simulink model "AUAV3_AND_SLUGS_SENSOR"  (Simulink 7.8)
settings: Solver=FixedStepDiscrete  StartTime=0.0  StopTime=10.0  FixedStep=T  RelTol=1e-3
PreLoadFcn:
  | T = 0.0025;
  | MavlinkBus;
  | 
  | % Baro Altitude Computation
  | % =========================
  | basePressure = 98192.64;
  | baseTemp = 288.215;
  | lapseRate = -0.00198122;
  | baseHeight = 0;
  | 
  | mcuInit
values from neighbouring files (symbols this model uses):
  apSampleTime = 0.01    [mcuInit.m]
  mavlink_gps_raw_int_t = Simulink.Bus    [MavlinkBus.m]    (also in MavlinkBusMarcello.m)
  mavlink_raw_imu_t = Simulink.Bus    [MavlinkBus.m]    (also in MavlinkBusMarcello.m)
  mavlink_scaled_pressure_t = Simulink.Bus    [MavlinkBus.m]    (also in MavlinkBusMarcello.m)
  mavlink_sys_status_t = Simulink.Bus    [MavlinkBus.m]    (also in MavlinkBusMarcello.m)
undefined symbols (not defined in the file or in its folder): A0, A14, A15, A2, A3, A5, A6, B0, barAdjust, baroCutTemp, baroOffset, baroScale, barTGain1, barTGain2, barTMean1, barTMean2, cubeAccelGain16405, cubeGyroGain16405, cubeMagGain16405, D0, D11, D8, G0, G15, gaind, IC1max, lowRateSensorCutoff, mainSensorCutoff, Max, maxDynPressure, ms, OC1max, P112, P127, P16, P21, P30, P31, P64, P72, P75, P80, P82, P83, Pin, pitAdjust, pitCutTemp, pitotOffset, pitotScale, pitTGain1, pitTGain2, pitTMean1, pitTMean2, polesd, powerOffset, powerScale, pressureSensorCutoff, Resol, tempOffset, tempScale ... (+5)
libraries: MCHP_Blockset x56, simulink x21, aerolibconvert2 x2
(part 4 of 5)

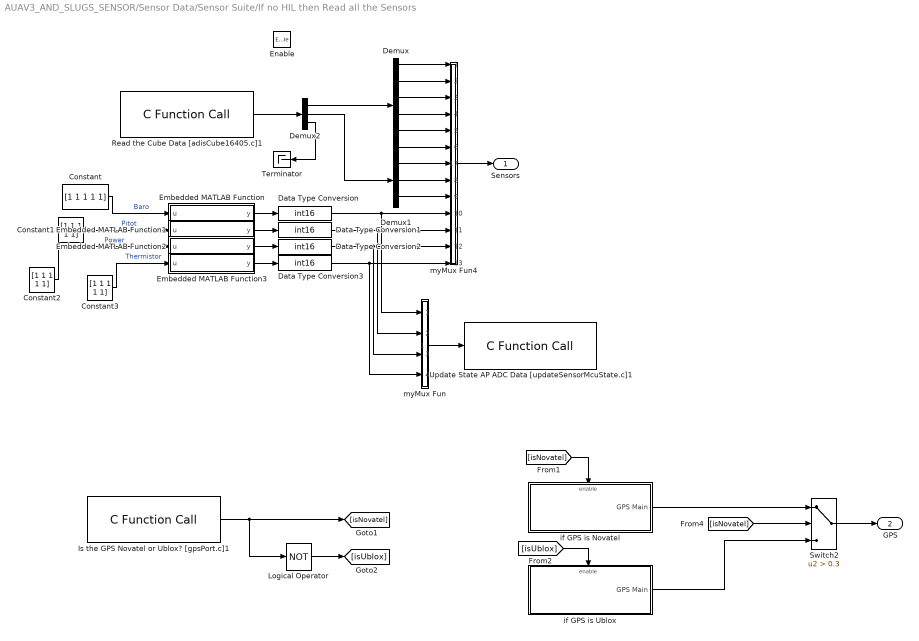
== system AUAV3_AND_SLUGS_SENSOR/Sensor Data/Sensor Suite/If no HIL then Read all the Sensors ==
  Enable : EnablePort
  Constant{,1..3} (4 alike) : Constant  Value=[1 1 1 1 1]
  Data Type Conversion{,1..3} (4 alike) : DataTypeConversion  OutDataTypeStr=int16
  Demux : Demux  Outputs=6
  Demux1 : Demux  Outputs=3
  Demux2 : Demux  Outputs=[6 3 1]
  Embedded MATLAB Function : MATLAB Function  TreatAsAtomicUnit=on
  Embedded MATLAB Function1 : MATLAB Function  TreatAsAtomicUnit=on
  Embedded MATLAB Function2 : MATLAB Function  TreatAsAtomicUnit=on
  Embedded MATLAB Function3 : MATLAB Function  TreatAsAtomicUnit=on
  Is the GPS Novatel or Ublox? [gpsPort.c]1 : MCHP_Blockset/User Functions/C Function Call  ParseFilesChkbx=off  ListFunctions1=Custom Function  Function1=extern uint8_T isGPSNovatel();  AddHeaderDeclaration=off  Function1Type=when block is updated (default)  FctReturnBlockOut=off  Fct1BlockOut=y[2]  DataCollected=0  ORDERING=Output  SampleTime=.01  MCHP_MASTERLINK=|  PinDigitalInput=[]  PinDigitalOutput=[]  PinAnalogInput=[]
      | AUAV3_AND_SLUGS_SENSOR/Microchip Master
      | AUAV V3 Board
      | Busy Flag on D2 (RA6)
  Logical Operator : Logic  Operator=NOT  AllPortsSameDT=off  OutDataTypeStr=boolean
  Read the Cube Data [adisCube16405.c]1 : MCHP_Blockset/User Functions/C Function Call  ParseFilesChkbx=off  ListFunctions1=Custom Function  Function1=extern void getCubeData(int16_T* y1);  AddHeaderDeclaration=off  Function1Type=when block is updated (default)  FctReturnBlockOut=off  Fct1BlockOut=y1[10]  ORDERING=None  SampleTime=.01  MCHP_MASTERLINK=|  PinDigitalInput=[]  PinDigitalOutput=[]  PinAnalogInput=[]
      | AUAV3_AND_SLUGS_SENSOR/Microchip Master
      | AUAV V3 Board
      | Busy Flag on D2 (RA6)
  Switch2 : Switch  Criteria=u2 > Threshold  Threshold=0.3  ZeroCross=off
  Terminator : Terminator
  Update State AP ADC Data [updateSensorMcuState.c]1 : MCHP_Blockset/User Functions/C Function Call  ParseFilesChkbx=off  ListFunctions1=Custom Function  Function1=extern void updateRawADCData(int16_T* u1);  AddHeaderDeclaration=off  Function1Type=when block is updated (default)  Fct1BlockIn=u1  FctReturnBlockOut=off  Fct1BlockOut=u1  DataCollected=0  ORDERING=None  SampleTime=.01  MCHP_MASTERLINK=|  PinDigitalInput=[]  PinDigitalOutput=[]  PinAnalogInput=[]
      | AUAV3_AND_SLUGS_SENSOR/Microchip Master
      | AUAV V3 Board
      | Busy Flag on D2 (RA6)
  if GPS is Novatel : Subsystem
  if GPS is Ublox : Subsystem
  myMux Fun : MATLAB Function  TreatAsAtomicUnit=on
  myMux Fun4 : MATLAB Function  TreatAsAtomicUnit=on
  Sensors : Outport
  GPS : Outport  Port=2
  wires:
  myMux Fun4/1(y) -> Sensors/1
  Demux2/1 -> Demux/1
  Demux/1 -> myMux Fun4/1(u1)
  Demux/2 -> myMux Fun4/2(u2)
  Demux/3 -> myMux Fun4/3(u3)
  Demux/4 -> myMux Fun4/4(u4)
  Demux/5 -> myMux Fun4/5(u5)
  Demux/6 -> myMux Fun4/6(u6)
  Demux1/1 -> myMux Fun4/7(u7)
  Demux1/2 -> myMux Fun4/8(u8)
  Demux1/3 -> myMux Fun4/9(u9)
  Constant/1 -> Embedded MATLAB Function/1(u)  "Baro"
  Constant1/1 -> Embedded MATLAB Function1/1(u)  "Pitot"
  Constant2/1 -> Embedded MATLAB Function2/1(u)  "Power"
  Constant3/1 -> Embedded MATLAB Function3/1(u)  "Thermistor"
  myMux Fun/1(y) -> Update State AP ADC Data [updateSensorMcuState.c]1/1
  Data Type Conversion/1 -> myMux Fun4/10(u10), myMux Fun/1(u1)
  Data Type Conversion1/1 -> myMux Fun4/11(u11), myMux Fun/2(u2)
  Data Type Conversion2/1 -> myMux Fun4/12(u12), myMux Fun/3(u3)
  Data Type Conversion3/1 -> myMux Fun4/13(u13), myMux Fun/4(u4)
  Embedded MATLAB Function/1(y) -> Data Type Conversion/1
  Embedded MATLAB Function1/1(y) -> Data Type Conversion1/1
  Embedded MATLAB Function2/1(y) -> Data Type Conversion2/1
  Embedded MATLAB Function3/1(y) -> Data Type Conversion3/1
  Read the Cube Data [adisCube16405.c]1/1 -> Demux2/1
  Demux2/3 -> Terminator/1
  Demux2/2 -> Demux1/1
  [isNovatel] -> Switch2/2
  Switch2/1 -> GPS/1
  Is the GPS Novatel or Ublox? [gpsPort.c]1/1 -> [isNovatel], Logical Operator/1
  if GPS is Novatel/1(GPS Main) -> Switch2/1
  Logical Operator/1 -> [isUblox]
  [isNovatel] -> if GPS is Novatel/Enable
  [isUblox] -> if GPS is Ublox/Enable
  if GPS is Ublox/1(GPS Main) -> Switch2/3

== system AUAV3_AND_SLUGS_SENSOR/Sensor Data/Sensor Suite/If no HIL then update Air Data ==
  AirData : Inport
  Enable : EnablePort
  Demux : Demux  Outputs=[1 2]
  Terminator : Terminator
  Update the Air Calibrated Data [updateSensorMcuState.c]1 : MCHP_Blockset/User Functions/C Function Call  ParseFilesChkbx=off  ListFunctions1=Custom Function  Function1=extern void updateAirData(real32_T* u1);  AddHeaderDeclaration=off  Function1Type=when block is updated (default)  FctReturnBlockOut=off  DataCollected=0  ORDERING=None  SampleTime=.01  MCHP_MASTERLINK=|  PinDigitalInput=[]  PinDigitalOutput=[]  PinAnalogInput=[]
      | AUAV3_AND_SLUGS_SENSOR/Microchip Master
      | AUAV V3 Board
      | Busy Flag on D2 (RA6)
  Out1 : Outport
  wires:
  AirData/1 -> Demux/1, Update the Air Calibrated Data [updateSensorMcuState.c]1/1
  Demux/1 -> Out1/1
  Demux/2 -> Terminator/1

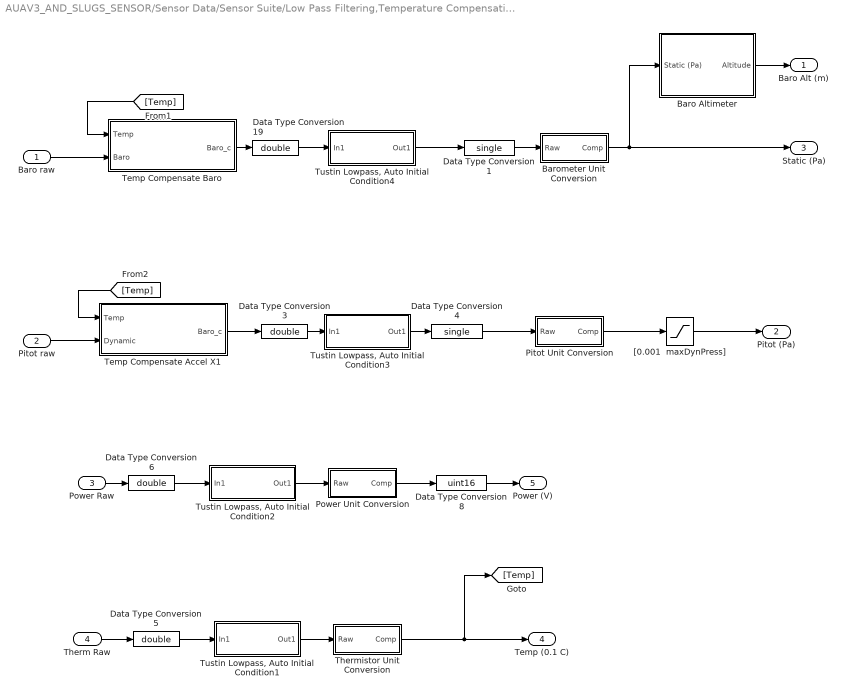
== system AUAV3_AND_SLUGS_SENSOR/Sensor Data/Sensor Suite/Low Pass Filtering,Temperature Compensation and Calibration ==
  Baro raw : Inport
  Pitot raw : Inport  Port=2
  Power Raw : Inport  Port=3
  Therm Raw : Inport  Port=4
  Baro Altimeter : Subsystem
  Barometer Unit Conversion : Subsystem  mask{bias=baroOffset, gains=baroScale}
      mask prompts: bias "Initial Bias"; gains "Initial Gains"
      mask help: Convert Analog readings to units
  Data Type Conversion1 : DataTypeConversion  OutDataTypeStr=single
  Data Type Conversion{3,5..6,19} (4 alike) : DataTypeConversion  OutDataTypeStr=double
  Data Type Conversion4 : DataTypeConversion  OutDataTypeStr=single
  Data Type Conversion8 : DataTypeConversion  OutDataTypeStr=uint16
  Pitot Unit Conversion : Subsystem  mask{bias=pitotOffset, gains=pitotScale}
      mask prompts: bias "Initial Bias"; gains "Initial Gains"
      mask help: Convert Analog readings to units
  Power Unit Conversion : Subsystem  mask{bias=powerOffset, gains=powerScale}
      mask prompts: bias "Initial Bias"; gains "Initial Gains"
      mask help: Convert Analog readings to units
  Temp Compensate Accel X1 : Subsystem
  Temp Compensate Baro : Subsystem
  Thermistor Unit Conversion : Subsystem  mask{bias=tempOffset, gains=tempScale}
      mask prompts: bias "Initial Bias"; gains "Initial Gains"
      mask help: Convert Analog readings to units
  "Tustin Lowpass, Auto Initial Condition1" : Subsystem  mask(Tustin1stOrderLowpassAutoInitialCondition){f=lowRateSensorCutoff, T=apSampleTime}
      mask prompts: f "Lowpass Frequency"; T "Sample Time"
      mask help: Takes a 3db rolloff frequency (in Hz, NOT radians/s) and a sample time. Performs a symbolic Tustin conversion and implements in a discrete filter. The initial output of the filter is set by the first sample.
      mask Help: Enter the desired 3db rolloff frequency in Hz and the sample time. Initial conditions are sampled automatically.
      mask Display: fprintf('%.2f Hz lowpass',f)
  "Tustin Lowpass, Auto Initial Condition2" : Subsystem  mask(Tustin1stOrderLowpassAutoInitialCondition){f=lowRateSensorCutoff, T=apSampleTime}
      mask prompts: f "Lowpass Frequency"; T "Sample Time"
      mask help: Takes a 3db rolloff frequency (in Hz, NOT radians/s) and a sample time. Performs a symbolic Tustin conversion and implements in a discrete filter. The initial output of the filter is set by the first sample.
      mask Help: Enter the desired 3db rolloff frequency in Hz and the sample time. Initial conditions are sampled automatically.
      mask Display: fprintf('%.2f Hz lowpass',f)
  "Tustin Lowpass, Auto Initial Condition3" : Subsystem  mask(Tustin1stOrderLowpassAutoInitialCondition){f=pressureSensorCutoff, T=apSampleTime}
      mask prompts: f "Lowpass Frequency"; T "Sample Time"
      mask help: Takes a 3db rolloff frequency (in Hz, NOT radians/s) and a sample time. Performs a symbolic Tustin conversion and implements in a discrete filter. The initial output of the filter is set by the first sample.
      mask Help: Enter the desired 3db rolloff frequency in Hz and the sample time. Initial conditions are sampled automatically.
      mask Display: fprintf('%.2f Hz lowpass',f)
  "Tustin Lowpass, Auto Initial Condition4" : Subsystem  mask(Tustin1stOrderLowpassAutoInitialCondition){f=pressureSensorCutoff, T=apSampleTime}
      mask prompts: f "Lowpass Frequency"; T "Sample Time"
      mask help: Takes a 3db rolloff frequency (in Hz, NOT radians/s) and a sample time. Performs a symbolic Tustin conversion and implements in a discrete filter. The initial output of the filter is set by the first sample.
      mask Help: Enter the desired 3db rolloff frequency in Hz and the sample time. Initial conditions are sampled automatically.
      mask Display: fprintf('%.2f Hz lowpass',f)
  "[0.001  maxDynPress]" : Saturate  UpperLimit=maxDynPressure  LowerLimit=0.001
  Baro Alt (m) : Outport
  Pitot (Pa) : Outport  Port=2
  Static (Pa) : Outport  Port=3
  Temp (0.1 C) : Outport  Port=4
  Power (V) : Outport  Port=5
  wires:
  "Tustin Lowpass, Auto Initial Condition1"/1(Out1) -> Thermistor Unit Conversion/1(Raw)
  "[0.001  maxDynPress]"/1 -> Pitot (Pa)/1
  Data Type Conversion19/1 -> "Tustin Lowpass, Auto Initial Condition4"/1(In1)
  Data Type Conversion3/1 -> "Tustin Lowpass, Auto Initial Condition3"/1(In1)
  "Tustin Lowpass, Auto Initial Condition3"/1(Out1) -> Data Type Conversion4/1
  Data Type Conversion5/1 -> "Tustin Lowpass, Auto Initial Condition1"/1(In1)
  Therm Raw/1 -> Data Type Conversion5/1
  Barometer Unit Conversion/1(Comp) -> Static (Pa)/1, Baro Altimeter/1(Static (Pa))
  Data Type Conversion4/1 -> Pitot Unit Conversion/1(Raw)
  "Tustin Lowpass, Auto Initial Condition4"/1(Out1) -> Data Type Conversion1/1
  Data Type Conversion1/1 -> Barometer Unit Conversion/1(Raw)
  Thermistor Unit Conversion/1(Comp) -> Temp (0.1 C)/1, [Temp]
  Data Type Conversion6/1 -> "Tustin Lowpass, Auto Initial Condition2"/1(In1)
  Power Raw/1 -> Data Type Conversion6/1
  "Tustin Lowpass, Auto Initial Condition2"/1(Out1) -> Power Unit Conversion/1(Raw)
  Data Type Conversion8/1 -> Power (V)/1
  Baro Altimeter/1(Altitude) -> Baro Alt (m)/1
  Pitot Unit Conversion/1(Comp) -> "[0.001  maxDynPress]"/1
  Power Unit Conversion/1(Comp) -> Data Type Conversion8/1
  Temp Compensate Baro/1(Baro_c) -> Data Type Conversion19/1
  [Temp] -> Temp Compensate Baro/1(Temp)
  Baro raw/1 -> Temp Compensate Baro/2(Baro)
  [Temp] -> Temp Compensate Accel X1/1(Temp)
  Pitot raw/1 -> Temp Compensate Accel X1/2(Dynamic)
  Temp Compensate Accel X1/1(Baro_c) -> Data Type Conversion3/1

== system AUAV3_AND_SLUGS_SENSOR/Read Barometer BMP180/Baro Altimeter/Initial Baro Bias/Low Pass8 ==
  In1 : Inport
  Discrete Zero-Pole : DiscreteZeroPole  Zeros=zerosd  Poles=polesd  Gain=gaind  SampleTime=SampleTime
  Out1 : Outport
  wires:
  Discrete Zero-Pole/1 -> Out1/1
  In1/1 -> Discrete Zero-Pole/1

== system AUAV3_AND_SLUGS_SENSOR/Sensor Data/Sensor Suite/ADIS16405 Signal Cond /3D Tustin Lowpass, Auto Initial Condition ==
  In1 : Inport
  Constant : Constant  Value=T
  Constant1 : Constant  Value=f
  Constant2 : Constant  Value=T
  Constant3 : Constant  Value=f
  Constant4 : Constant  Value=T
  Constant5 : Constant  Value=f
  Demux : Demux  Outputs=3
  Embedded MATLAB Function : MATLAB Function  TreatAsAtomicUnit=on
  Embedded MATLAB Function1 : MATLAB Function  TreatAsAtomicUnit=on
  Embedded MATLAB Function2 : MATLAB Function  TreatAsAtomicUnit=on
  myMux Fun : MATLAB Function  TreatAsAtomicUnit=on
  Out1 : Outport
  wires:
  myMux Fun/1(y) -> Out1/1
  In1/1 -> Demux/1
  Embedded MATLAB Function1/1(y) -> myMux Fun/2(u2)
  Demux/3 -> Embedded MATLAB Function2/1(u)
  Demux/2 -> Embedded MATLAB Function1/1(u)
  Demux/1 -> Embedded MATLAB Function/1(u)
  Embedded MATLAB Function2/1(y) -> myMux Fun/3(u3)
  Constant5/1 -> Embedded MATLAB Function2/3(f)
  Constant4/1 -> Embedded MATLAB Function2/2(T)
  Constant3/1 -> Embedded MATLAB Function1/3(f)
  Constant2/1 -> Embedded MATLAB Function1/2(T)
  Embedded MATLAB Function/1(y) -> myMux Fun/1(u1)
  Constant1/1 -> Embedded MATLAB Function/3(f)
  Constant/1 -> Embedded MATLAB Function/2(T)

== system AUAV3_AND_SLUGS_SENSOR/Sensor Data/Sensor Suite/ADIS16405 Signal Cond /3D Tustin Lowpass, Auto Initial Condition1 ==
  In1 : Inport
  Constant : Constant  Value=T
  Constant1 : Constant  Value=f
  Constant2 : Constant  Value=T
  Constant3 : Constant  Value=f
  Constant4 : Constant  Value=T
  Constant5 : Constant  Value=f
  Demux : Demux  Outputs=3
  Embedded MATLAB Function : MATLAB Function  TreatAsAtomicUnit=on
  Embedded MATLAB Function1 : MATLAB Function  TreatAsAtomicUnit=on
  Embedded MATLAB Function2 : MATLAB Function  TreatAsAtomicUnit=on
  myMux Fun : MATLAB Function  TreatAsAtomicUnit=on
  Out1 : Outport
  wires:
  myMux Fun/1(y) -> Out1/1
  In1/1 -> Demux/1
  Embedded MATLAB Function1/1(y) -> myMux Fun/2(u2)
  Demux/3 -> Embedded MATLAB Function2/1(u)
  Demux/2 -> Embedded MATLAB Function1/1(u)
  Demux/1 -> Embedded MATLAB Function/1(u)
  Embedded MATLAB Function2/1(y) -> myMux Fun/3(u3)
  Constant5/1 -> Embedded MATLAB Function2/3(f)
  Constant4/1 -> Embedded MATLAB Function2/2(T)
  Constant3/1 -> Embedded MATLAB Function1/3(f)
  Constant2/1 -> Embedded MATLAB Function1/2(T)
  Embedded MATLAB Function/1(y) -> myMux Fun/1(u1)
  Constant1/1 -> Embedded MATLAB Function/3(f)
  Constant/1 -> Embedded MATLAB Function/2(T)

== system AUAV3_AND_SLUGS_SENSOR/Sensor Data/Sensor Suite/ADIS16405 Signal Cond /3D Tustin Lowpass, Auto Initial Condition2 ==
  In1 : Inport
  Constant : Constant  Value=T
  Constant1 : Constant  Value=f
  Constant2 : Constant  Value=T
  Constant3 : Constant  Value=f
  Constant4 : Constant  Value=T
  Constant5 : Constant  Value=f
  Demux : Demux  Outputs=3
  Embedded MATLAB Function : MATLAB Function  TreatAsAtomicUnit=on
  Embedded MATLAB Function1 : MATLAB Function  TreatAsAtomicUnit=on
  Embedded MATLAB Function2 : MATLAB Function  TreatAsAtomicUnit=on
  myMux Fun : MATLAB Function  TreatAsAtomicUnit=on
  Out1 : Outport
  wires:
  Constant/1 -> Embedded MATLAB Function/2(T)
  Constant1/1 -> Embedded MATLAB Function/3(f)
  Embedded MATLAB Function/1(y) -> myMux Fun/1(u1)
  Constant2/1 -> Embedded MATLAB Function1/2(T)
  Constant3/1 -> Embedded MATLAB Function1/3(f)
  Constant4/1 -> Embedded MATLAB Function2/2(T)
  Constant5/1 -> Embedded MATLAB Function2/3(f)
  Embedded MATLAB Function2/1(y) -> myMux Fun/3(u3)
  Demux/1 -> Embedded MATLAB Function/1(u)
  Demux/2 -> Embedded MATLAB Function1/1(u)
  Demux/3 -> Embedded MATLAB Function2/1(u)
  Embedded MATLAB Function1/1(y) -> myMux Fun/2(u2)
  In1/1 -> Demux/1
  myMux Fun/1(y) -> Out1/1

== system AUAV3_AND_SLUGS_SENSOR/Sensor Data/Sensor Suite/ADIS16405 Signal Cond /Rotate Cube Axis ==
  Raw : Inport
  Selector : Selector  InputPortWidth=3  IndexOptions=Index vector (dialog)  Indices=[2 1 3]  OutputSizes=1
  "[ -1 -1 -1]" : Gain  Gain=[-1 -1 -1]
  Rotated : Outport
  wires:
  Selector/1 -> "[ -1 -1 -1]"/1
  Raw/1 -> Selector/1
  "[ -1 -1 -1]"/1 -> Rotated/1

== system AUAV3_AND_SLUGS_SENSOR/Sensor Data/Sensor Suite/ADIS16405 Signal Cond /Rotate Cube Axis  ==
  Raw : Inport
  Selector : Selector  InputPortWidth=3  IndexOptions=Index vector (dialog)  Indices=[2 1 3]  OutputSizes=1
  Rotated : Outport
  wires:
  Raw/1 -> Selector/1
  Selector/1 -> Rotated/1

== system AUAV3_AND_SLUGS_SENSOR/Sensor Data/Sensor Suite/ADIS16405 Signal Cond /Rotate Cube Axis   ==
  Raw : Inport
  Selector : Selector  InputPortWidth=3  IndexOptions=Index vector (dialog)  Indices=[2 1 3]  OutputSizes=1
  "[ -1 -1 -1]" : Gain  Gain=[-1 -1 -1]
  Rotated : Outport
  wires:
  "[ -1 -1 -1]"/1 -> Rotated/1
  Raw/1 -> Selector/1
  Selector/1 -> "[ -1 -1 -1]"/1

== system AUAV3_AND_SLUGS_SENSOR/Sensor Data/Sensor Suite/If no HIL then Read all the Sensors/if GPS is Novatel ==
  Enable : EnablePort
  Parse the GPS RAW Data [gps.c/novatel.c]1 : MCHP_Blockset/User Functions/C Function Call  ParseFilesChkbx=off  ListFunctions1=Custom Function  Function1=extern void gpsParse(uint8_T* u1);  AddHeaderDeclaration=off  Function1Type=when block is updated (default)  Fct1BlockIn=u1  FctReturnBlockOut=off  Fct1BlockOut=u1*  DataCollected=0  ORDERING=None  SampleTime=.01  MCHP_MASTERLINK=|  PinDigitalInput=[]  PinDigitalOutput=[]  PinAnalogInput=[]
      | AUAV3_AND_SLUGS_SENSOR/Microchip Master
      | AUAV V3 Board
      | Busy Flag on D2 (RA6)
  Produce the GPS Main Data and update the AP State (lat lon hei cog sog) [gps.c/novatel.c]1 : MCHP_Blockset/User Functions/C Function Call  ParseFilesChkbx=off  ListFunctions1=Custom Function  Function1=extern void getGpsMainData(real32_T* y1);  AddHeaderDeclaration=off  Function1Type=when block is updated (default)  FctReturnBlockOut=off  Fct1BlockOut=y1  DataCollected=0  ORDERING=None  SampleTime=.01  MCHP_MASTERLINK=|  PinDigitalInput=[]  PinDigitalOutput=[]  PinAnalogInput=[]
      | AUAV3_AND_SLUGS_SENSOR/Microchip Master
      | AUAV V3 Board
      | Busy Flag on D2 (RA6)
  Read the Raw Data from GPS [gpsPort.c]1 : MCHP_Blockset/User Functions/C Function Call  ParseFilesChkbx=off  ListFunctions1=Custom Function  Function1=extern void getGPSRawData(uint8_T* y1);  AddHeaderDeclaration=off  Function1Type=when block is updated (default)  FctReturnBlockOut=off  Fct1BlockOut=y1  DataCollected=0  ORDERING=None  SampleTime=.01  MCHP_MASTERLINK=|  PinDigitalInput=[]  PinDigitalOutput=[]  PinAnalogInput=[]
      | AUAV3_AND_SLUGS_SENSOR/Microchip Master
      | AUAV V3 Board
      | Busy Flag on D2 (RA6)
  GPS Main : Outport
  wires:
  Produce the GPS Main Data and update the AP State (lat lon hei cog sog) [gps.c/novatel.c]1/1 -> GPS Main/1
  Read the Raw Data from GPS [gpsPort.c]1/1 -> Parse the GPS RAW Data [gps.c/novatel.c]1/1

== system AUAV3_AND_SLUGS_SENSOR/Sensor Data/Sensor Suite/If no HIL then Read all the Sensors/if GPS is Ublox ==
  Enable : EnablePort
  Produce the GPS Main Data and update the AP State (lat lon hei cog sog) [gpsUblox.c]1 : MCHP_Blockset/User Functions/C Function Call  ParseFilesChkbx=off  ListFunctions1=Custom Function  Function1=extern void getGpsUbloxMainData(real32_T* y1);  AddHeaderDeclaration=off  Function1Type=when block is updated (default)  FctReturnBlockOut=off  Fct1BlockOut=y1  DataCollected=0  ORDERING=None  SampleTime=.01  MCHP_MASTERLINK=|  PinDigitalInput=[]  PinDigitalOutput=[]  PinAnalogInput=[]
      | AUAV3_AND_SLUGS_SENSOR/Microchip Master
      | AUAV V3 Board
      | Busy Flag on D2 (RA6)
  GPS Main : Outport
  wires:
  Produce the GPS Main Data and update the AP State (lat lon hei cog sog) [gpsUblox.c]1/1 -> GPS Main/1

== system AUAV3_AND_SLUGS_SENSOR/Sensor Data/Sensor Suite/Low Pass Filtering,Temperature Compensation and Calibration/Baro Altimeter ==
  Static (Pa) : Inport
  Compute Barometric Height : Subsystem  mask{baseTemp=baseTemp, LapseRate=lapseRate}
      mask prompts: baseTemp "Base Station Temperature (K)"; LapseRate "Lapse Rate (C/ft)"
      mask help:
      | Produces Altitude in meters from Barometric Pressure in Pascals. Altitude is valid from MSL to 6000 ft.
      |
      | The method implemented here was developed by Ren Curry
  Enabled Subsystem : Subsystem  TreatAsAtomicUnit=on
  Enables/Disables the Computation of  initial Baro Bias : MATLAB Function  TreatAsAtomicUnit=on
  GS Height : Subsystem
  Initial Baro Bias : Subsystem  TreatAsAtomicUnit=on
  Logical Operator : Logic  Operator=NOT  AllPortsSameDT=off  OutDataTypeStr=boolean
  Sum1 : Sum  Inputs=++|  OutDataTypeStr=single
  Zero Out Height : Subsystem  TreatAsAtomicUnit=on
  Altitude : Outport
  wires:
  Compute Barometric Height/1("Altitude, m") -> Zero Out Height/2(Computed Height), Sum1/2
  Static (Pa)/1 -> Initial Baro Bias/1(Baro (Pa)), Compute Barometric Height/3(Baro (Pa))
  Enables/Disables the Computation of  initial Baro Bias/1(tOut) -> Initial Baro Bias/Enable, Zero Out Height/Enable, Logical Operator/1
  GS Height/1(GS Height) -> Compute Barometric Height/1(Base Height (m)), Zero Out Height/1(Base Height)
  Initial Baro Bias/1(Baro (Gnd)) -> Compute Barometric Height/2(Base Pressure (Pa))
  Zero Out Height/1(Height Offset) -> Sum1/1
  Logical Operator/1 -> Enabled Subsystem/Enable
  Sum1/1 -> Enabled Subsystem/1(In1)
  Enabled Subsystem/1(Out1) -> Altitude/1

== system AUAV3_AND_SLUGS_SENSOR/Sensor Data/Sensor Suite/Low Pass Filtering,Temperature Compensation and Calibration/Barometer Unit Conversion ==
  Raw : Inport
  Bias : Constant  Value=bias  OutDataTypeStr=single
  Divide : Product  OutDataTypeStr=single
  Gains : Constant  Value=gains  OutDataTypeStr=single
  Sum : Sum  Inputs=|++  OutDataTypeStr=single
  Comp : Outport
  wires:
  Bias/1 -> Sum/2
  Raw/1 -> Divide/2
  Gains/1 -> Divide/1
  Divide/1 -> Sum/1
  Sum/1 -> Comp/1

== system AUAV3_AND_SLUGS_SENSOR/Sensor Data/Sensor Suite/Low Pass Filtering,Temperature Compensation and Calibration/Pitot Unit Conversion ==
  Raw : Inport
  Bias : Constant  Value=bias  OutDataTypeStr=single
  Divide : Product  OutDataTypeStr=single
  Gains : Constant  Value=gains  OutDataTypeStr=single
  Sum : Sum  Inputs=|++  OutDataTypeStr=single
  Comp : Outport
  wires:
  Bias/1 -> Sum/2
  Raw/1 -> Divide/2
  Gains/1 -> Divide/1
  Divide/1 -> Sum/1
  Sum/1 -> Comp/1

== system AUAV3_AND_SLUGS_SENSOR/Sensor Data/Sensor Suite/Low Pass Filtering,Temperature Compensation and Calibration/Power Unit Conversion ==
  Raw : Inport
  Bias : Constant  Value=bias  OutDataTypeStr=single
  Divide : Product  OutDataTypeStr=single
  Gains : Constant  Value=gains  OutDataTypeStr=single
  Sum : Sum  Inputs=|++  OutDataTypeStr=single
  Comp : Outport
  wires:
  Bias/1 -> Sum/2
  Raw/1 -> Divide/2
  Gains/1 -> Divide/1
  Divide/1 -> Sum/1
  Sum/1 -> Comp/1

== system AUAV3_AND_SLUGS_SENSOR/Sensor Data/Sensor Suite/Low Pass Filtering,Temperature Compensation and Calibration/Temp Compensate Accel X1 ==
  Temp : Inport
  Dynamic : Inport  Port=2
  Compare To Constant : simulink/Logic and Bit Operations/Compare To Constant  relop=<  const=pitCutTemp  OutDataTypeStr=uint8  ZeroCross=off
  Display : Display
  Display2 : Display
  Hi Temp Compensation2 : Subsystem  mask{alpha=pitTGain2, tempMean=pitTMean2}
      mask prompts: alpha "Tempearature Coeficient (K_t)"; tempMean "Calibration Temperature Mean (T_avg)"
      mask help:
      | This block implements a temperature compensation. It implmements the following equation:
      |
      | M_tc = M_raw - K_t(T - T_avg)
  Lo Temp Compensation : Subsystem  mask{alpha=pitTGain1, tempMean=pitTMean1}
      mask prompts: alpha "Tempearature Coeficient (K_t)"; tempMean "Calibration Temperature Mean (T_avg)"
      mask help:
      | This block implements a temperature compensation. It implmements the following equation:
      |
      | M_tc = M_raw - K_t(T - T_avg)
  Logical Operator : Logic  Operator=NOT  AllPortsSameDT=off  OutDataTypeStr=boolean
  Merge : Merge
  Baro_c : Outport
  wires:
  Hi Temp Compensation2/1(Comp) -> Merge/1
  Logical Operator/1 -> Hi Temp Compensation2/Enable, Display2/1
  Merge/1 -> Baro_c/1, Display/1
  Dynamic/1 -> Lo Temp Compensation/1(Raw), Hi Temp Compensation2/1(Raw)
  Temp/1 -> Compare To Constant/1, Lo Temp Compensation/2(Temp Raw), Hi Temp Compensation2/2(Temp Raw)
  Compare To Constant/1 -> Lo Temp Compensation/Enable, Logical Operator/1
  Lo Temp Compensation/1(Comp) -> Merge/2

== system AUAV3_AND_SLUGS_SENSOR/Sensor Data/Sensor Suite/Low Pass Filtering,Temperature Compensation and Calibration/Temp Compensate Baro ==
  Temp : Inport
  Baro : Inport  Port=2
  Compare To Constant : simulink/Logic and Bit Operations/Compare To Constant  relop=<  const=baroCutTemp  OutDataTypeStr=uint8  ZeroCross=off
  Hi Temp Compensation : Subsystem  mask{alpha=barTGain2, tempMean=barTMean2}
      mask prompts: alpha "Tempearature Coeficient (K_t)"; tempMean "Calibration Temperature Mean (T_avg)"
      mask help:
      | This block implements a temperature compensation. It implmements the following equation:
      |
      | M_tc = M_raw - K_t(T - T_avg)
  Lo Temp Compensation : Subsystem  mask{alpha=barTGain1, tempMean=barTMean1}
      mask prompts: alpha "Tempearature Coeficient (K_t)"; tempMean "Calibration Temperature Mean (T_avg)"
      mask help:
      | This block implements a temperature compensation. It implmements the following equation:
      |
      | M_tc = M_raw - K_t(T - T_avg)
  Logical Operator : Logic  Operator=NOT  AllPortsSameDT=off  OutDataTypeStr=boolean
  Merge : Merge
  Baro_c : Outport
  wires:
  Compare To Constant/1 -> Logical Operator/1, Lo Temp Compensation/Enable
  Temp/1 -> Compare To Constant/1, Hi Temp Compensation/2(Temp Raw), Lo Temp Compensation/2(Temp Raw)
  Baro/1 -> Hi Temp Compensation/1(Raw), Lo Temp Compensation/1(Raw)
  Lo Temp Compensation/1(Comp) -> Merge/2
  Merge/1 -> Baro_c/1
  Logical Operator/1 -> Hi Temp Compensation/Enable
  Hi Temp Compensation/1(Comp) -> Merge/1

== system AUAV3_AND_SLUGS_SENSOR/Sensor Data/Sensor Suite/Low Pass Filtering,Temperature Compensation and Calibration/Thermistor Unit Conversion ==
  Raw : Inport
  Bias : Constant  Value=bias  OutDataTypeStr=single
  Divide : Product  OutDataTypeStr=single
  Gains : Constant  Value=gains  OutDataTypeStr=single
  Sum : Sum  Inputs=|++  OutDataTypeStr=single
  Comp : Outport
  wires:
  Sum/1 -> Comp/1
  Divide/1 -> Sum/1
  Gains/1 -> Divide/1
  Raw/1 -> Divide/2
  Bias/1 -> Sum/2

== system AUAV3_AND_SLUGS_SENSOR/Sensor Data/Sensor Suite/Low Pass Filtering,Temperature Compensation and Calibration/Tustin Lowpass, Auto Initial Condition1 ==
  In1 : Inport
  Constant : Constant  Value=T
  Constant1 : Constant  Value=f
  Embedded MATLAB Function : MATLAB Function  TreatAsAtomicUnit=on
  Out1 : Outport
  wires:
  Constant/1 -> Embedded MATLAB Function/2(T)
  Constant1/1 -> Embedded MATLAB Function/3(f)
  Embedded MATLAB Function/1(y) -> Out1/1
  In1/1 -> Embedded MATLAB Function/1(u)

== system AUAV3_AND_SLUGS_SENSOR/Sensor Data/Sensor Suite/Low Pass Filtering,Temperature Compensation and Calibration/Tustin Lowpass, Auto Initial Condition2 ==
  In1 : Inport
  Constant : Constant  Value=T
  Constant1 : Constant  Value=f
  Embedded MATLAB Function : MATLAB Function  TreatAsAtomicUnit=on
  Out1 : Outport
  wires:
  In1/1 -> Embedded MATLAB Function/1(u)
  Embedded MATLAB Function/1(y) -> Out1/1
  Constant1/1 -> Embedded MATLAB Function/3(f)
  Constant/1 -> Embedded MATLAB Function/2(T)

== system AUAV3_AND_SLUGS_SENSOR/Sensor Data/Sensor Suite/Low Pass Filtering,Temperature Compensation and Calibration/Tustin Lowpass, Auto Initial Condition3 ==
  In1 : Inport
  Constant : Constant  Value=T
  Constant1 : Constant  Value=f
  Embedded MATLAB Function : MATLAB Function  TreatAsAtomicUnit=on
  Out1 : Outport
  wires:
  Constant/1 -> Embedded MATLAB Function/2(T)
  Constant1/1 -> Embedded MATLAB Function/3(f)
  Embedded MATLAB Function/1(y) -> Out1/1
  In1/1 -> Embedded MATLAB Function/1(u)

== system AUAV3_AND_SLUGS_SENSOR/Sensor Data/Sensor Suite/Low Pass Filtering,Temperature Compensation and Calibration/Tustin Lowpass, Auto Initial Condition4 ==
  In1 : Inport
  Constant : Constant  Value=T
  Constant1 : Constant  Value=f
  Embedded MATLAB Function : MATLAB Function  TreatAsAtomicUnit=on
  Out1 : Outport
  wires:
  In1/1 -> Embedded MATLAB Function/1(u)
  Embedded MATLAB Function/1(y) -> Out1/1
  Constant1/1 -> Embedded MATLAB Function/3(f)
  Constant/1 -> Embedded MATLAB Function/2(T)

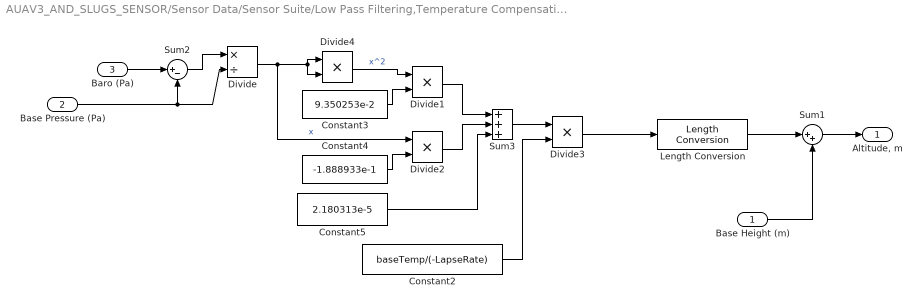
== system AUAV3_AND_SLUGS_SENSOR/Sensor Data/Sensor Suite/Low Pass Filtering,Temperature Compensation and Calibration/Baro Altimeter/Compute Barometric Height ==
  Base Height (m) : Inport
  Base Pressure (Pa) : Inport  Port=2
  Baro (Pa) : Inport  Port=3
  Constant2 : Constant  Value=baseTemp/(-LapseRate)  OutDataTypeStr=single
  Constant3 : Constant  Value=9.350253e-2  OutDataTypeStr=single
  Constant4 : Constant  Value=-1.888933e-1  OutDataTypeStr=single
  Constant5 : Constant  Value=2.180313e-5  OutDataTypeStr=single
  Divide : Product  Inputs=*/  OutDataTypeStr=single
  Divide{1..4} (4 alike) : Product  OutDataTypeStr=single
  Length Conversion : aerolibconvert2/Length Conversion  IU=ft  OU=m
  Sum1 : Sum  Inputs=|++  OutDataTypeStr=single
  Sum2 : Sum  Inputs=|+-  OutDataTypeStr=single
  Sum3 : Sum  Inputs=3  OutDataTypeStr=single
  "Altitude, m" : Outport
  wires:
  Length Conversion/1 -> Sum1/1
  Sum2/1 -> Divide/1
  Sum1/1 -> "Altitude, m"/1
  Divide3/1 -> Length Conversion/1
  Constant2/1 -> Divide3/2
  Sum3/1 -> Divide3/1
  Constant5/1 -> Sum3/3
  Divide2/1 -> Sum3/2
  Divide1/1 -> Sum3/1
  Constant4/1 -> Divide2/2
  Constant3/1 -> Divide1/2
  Divide4/1 -> Divide1/1  "x^2"
  Divide/1 -> Divide2/1, Divide4/1, Divide4/2  "x"
  Base Pressure (Pa)/1 -> Divide/2, Sum2/2
  Base Height (m)/1 -> Sum1/2
  Baro (Pa)/1 -> Sum2/1

== system AUAV3_AND_SLUGS_SENSOR/Sensor Data/Sensor Suite/Low Pass Filtering,Temperature Compensation and Calibration/Baro Altimeter/Enabled Subsystem ==
  In1 : Inport
  Enable : EnablePort
  Out1 : Outport  InitialOutput=baseHeight
  wires:
  In1/1 -> Out1/1

== system AUAV3_AND_SLUGS_SENSOR/Sensor Data/Sensor Suite/Low Pass Filtering,Temperature Compensation and Calibration/Baro Altimeter/GS Height ==
  Demux : Demux  Outputs=[1 2]
  Get the GS Location [updateSensorMCUState.c]1 : MCHP_Blockset/User Functions/C Function Call  ParseFilesChkbx=off  ListFunctions1=Custom Function  Function1=extern void getGSLocation(real32_T* y1);  AddHeaderDeclaration=off  Function1Type=when block is updated (default)  FctReturnBlockOut=off  Fct1BlockOut=y1  DataCollected=0  ORDERING=None  SampleTime=.01  MCHP_MASTERLINK=|  PinDigitalInput=[]  PinDigitalOutput=[]  PinAnalogInput=[]
      | AUAV3_AND_SLUGS_SENSOR/Microchip Master
      | AUAV V3 Board
      | Busy Flag on D2 (RA6)
  Terminator : Terminator
  GS Height : Outport
  wires:
  Get the GS Location [updateSensorMCUState.c]1/1 -> Demux/1
  Demux/2 -> Terminator/1
  Demux/1 -> GS Height/1

== system AUAV3_AND_SLUGS_SENSOR/Sensor Data/Sensor Suite/Low Pass Filtering,Temperature Compensation and Calibration/Baro Altimeter/Initial Baro Bias ==
  Baro (Pa) : Inport
  Enable : EnablePort
  Data Type Conversion : DataTypeConversion  OutDataTypeStr=double
  Data Type Conversion1 : DataTypeConversion  OutDataTypeStr=single
  Low Pass8 : Subsystem  mask(DiscretizedZeroPole){Zeros=[], Poles=[-3], Gain=3, AbsTol=auto, SampleTime=.01, method=tustin, Wc=1}
      mask prompts: Zeros "Zeros (enter in s-main:)"; Poles "Poles (enter in s-domain:)"; Gain "Gain (enter in s-domain:)"; AbsTol "Absolute tolerance:"; SampleTime "Sample time:"; Wc "Critical Frequency (Hz):"
      mask help: Continuous mask uses c2d to transform parameters onto the Discrete Zero-Pole block inside.
      mask init: same as AUAV3_AND_SLUGS_SENSOR/Read Barometer BMP180/Baro Altimeter/Initial Baro Bias/Low Pass8
      mask StyleString: edit,edit,edit,edit,edit,popup(zoh|foh|tustin|prewarp|matched),edit
      mask CallbackString: |||||hidecrit|
      mask Display:
      | droots(zeross,poless,gainss)
      | text( 0.5, 1.0, method, 'verticalAlignment','top')
  "[80k - 120k]" : Saturate  UpperLimit=120000  LowerLimit=80000
  Baro (Gnd) : Outport
  wires:
  Baro (Pa)/1 -> Data Type Conversion/1
  Low Pass8/1(Out1) -> Data Type Conversion1/1
  Data Type Conversion/1 -> Low Pass8/1(In1)
  Data Type Conversion1/1 -> "[80k - 120k]"/1
  "[80k - 120k]"/1 -> Baro (Gnd)/1

== system AUAV3_AND_SLUGS_SENSOR/Sensor Data/Sensor Suite/Low Pass Filtering,Temperature Compensation and Calibration/Baro Altimeter/Zero Out Height ==
  Base Height : Inport
  Computed Height : Inport  Port=2
  Enable : EnablePort
  Integer Delay : Delay  DelayLength=1  InitialCondition=0  InputProcessing=Inherited  SampleTime=.01
  Sum : Sum  Inputs=|+-  OutDataTypeStr=single
  Height Offset : Outport
  wires:
  Computed Height/1 -> Integer Delay/1
  Sum/1 -> Height Offset/1
  Integer Delay/1 -> Sum/2
  Base Height/1 -> Sum/1

== system AUAV3_AND_SLUGS_SENSOR/Sensor Data/Sensor Suite/Low Pass Filtering,Temperature Compensation and Calibration/Temp Compensate Accel X1/Hi Temp Compensation2 ==
  Raw : Inport
  Temp Raw : Inport  Port=2
  Enable : EnablePort
  Divide1 : Product  OutDataTypeStr=single
  Mean Temperature for Calibration : Constant  Value=tempMean  OutDataTypeStr=single
  Sum1 : Sum  Inputs=|+-  OutDataTypeStr=single
  Sum2 : Sum  Inputs=|+-  OutDataTypeStr=single
  gains : Constant  Value=alpha  OutDataTypeStr=single
  Comp : Outport
  wires:
  Mean Temperature for Calibration/1 -> Sum1/2
  Raw/1 -> Sum2/1
  Temp Raw/1 -> Sum1/1
  Sum1/1 -> Divide1/2
  gains/1 -> Divide1/1
  Divide1/1 -> Sum2/2
  Sum2/1 -> Comp/1

== system AUAV3_AND_SLUGS_SENSOR/Sensor Data/Sensor Suite/Low Pass Filtering,Temperature Compensation and Calibration/Temp Compensate Accel X1/Lo Temp Compensation ==
  Raw : Inport
  Temp Raw : Inport  Port=2
  Enable : EnablePort
  Add : Sum  OutDataTypeStr=single
  Constant : Constant  Value=pitAdjust  OutDataTypeStr=single
  Divide1 : Product  OutDataTypeStr=single
  Mean Temperature for Calibration : Constant  Value=tempMean  OutDataTypeStr=single
  Sum1 : Sum  Inputs=|+-  OutDataTypeStr=single
  Sum2 : Sum  Inputs=|+-  OutDataTypeStr=single
  gains : Constant  Value=alpha  OutDataTypeStr=single
  Comp : Outport
  wires:
  Add/1 -> Comp/1
  Constant/1 -> Add/2
  Sum2/1 -> Add/1
  Divide1/1 -> Sum2/2
  gains/1 -> Divide1/1
  Sum1/1 -> Divide1/2
  Temp Raw/1 -> Sum1/1
  Raw/1 -> Sum2/1
  Mean Temperature for Calibration/1 -> Sum1/2

== system AUAV3_AND_SLUGS_SENSOR/Sensor Data/Sensor Suite/Low Pass Filtering,Temperature Compensation and Calibration/Temp Compensate Baro/Hi Temp Compensation ==
  Raw : Inport
  Temp Raw : Inport  Port=2
  Enable : EnablePort
  Add : Sum  OutDataTypeStr=single
  Constant : Constant  Value=barAdjust  OutDataTypeStr=single
  Divide1 : Product  OutDataTypeStr=single
  Mean Temperature for Calibration : Constant  Value=tempMean  OutDataTypeStr=single
  Sum1 : Sum  Inputs=|+-  OutDataTypeStr=single
  Sum2 : Sum  Inputs=|+-  OutDataTypeStr=single
  gains : Constant  Value=alpha  OutDataTypeStr=single
  Comp : Outport
  wires:
  Sum2/1 -> Add/2
  Add/1 -> Comp/1
  Constant/1 -> Add/1
  Divide1/1 -> Sum2/2
  gains/1 -> Divide1/1
  Sum1/1 -> Divide1/2
  Temp Raw/1 -> Sum1/1
  Raw/1 -> Sum2/1
  Mean Temperature for Calibration/1 -> Sum1/2

== system AUAV3_AND_SLUGS_SENSOR/Sensor Data/Sensor Suite/Low Pass Filtering,Temperature Compensation and Calibration/Temp Compensate Baro/Lo Temp Compensation ==
  Raw : Inport
  Temp Raw : Inport  Port=2
  Enable : EnablePort
  Divide1 : Product  OutDataTypeStr=single
  Mean Temperature for Calibration : Constant  Value=tempMean  OutDataTypeStr=single
  Sum1 : Sum  Inputs=|+-  OutDataTypeStr=single
  Sum2 : Sum  Inputs=|+-  OutDataTypeStr=single
  gains : Constant  Value=alpha  OutDataTypeStr=single
  Comp : Outport
  wires:
  Mean Temperature for Calibration/1 -> Sum1/2
  Raw/1 -> Sum2/1
  Temp Raw/1 -> Sum1/1
  Sum1/1 -> Divide1/2
  gains/1 -> Divide1/1
  Divide1/1 -> Sum2/2
  Sum2/1 -> Comp/1

== system AUAV3_AND_SLUGS_SENSOR/Sensor Data/Sensor Suite/Low Pass Filtering,Temperature Compensation and Calibration/Baro Altimeter/Initial Baro Bias/Low Pass8 ==
  In1 : Inport
  Discrete Zero-Pole : DiscreteZeroPole  Zeros=zerosd  Poles=polesd  Gain=gaind  SampleTime=SampleTime
  Out1 : Outport
  wires:
  In1/1 -> Discrete Zero-Pole/1
  Discrete Zero-Pole/1 -> Out1/1

== matlab function Sensor Data/Sensor Suite/myMux Fun ==
  data: u1 input double; y output double; u2 input double; u3 input double
function y = myMux3(u1, u2, u3)
% This block supports an embeddable subset of the MATLAB language.
% See the help menu for details. 

y = [u1(1); u2(1); u3(1)];

== matlab function Sensor Data/Sensor Suite/ADIS16405 Signal Cond /3D Tustin Lowpass, Auto Initial Condition2/Embedded MATLAB Function ==
  data: u input double; y output double; T input double; f input double
function y = fcn(u,T,f)
% This block supports an embeddable subset of the MATLAB language.
% See the help menu for details. 

persistent a
persistent b
persistent y_km1
persistent u_km1
if isempty(a)
    %tf = [T*omega/(2+T*omega) T*omega/(2+T*omega)],[1 (T*omega-2)/(T*omega+2)]
    %tf = [a a],[1 -b]
    omega = 2*pi*f;
    a=T*omega/(2+T*omega);
    b=-(T*omega-2)/(T*omega+2);
    y_km1=u;
    u_km1=u;
end

y = a*(u+u_km1)+b*y_km1;
y_km1=y;
u_km1=u;

== matlab function Sensor Data/Sensor Suite/ADIS16405 Signal Cond /3D Tustin Lowpass, Auto Initial Condition2/Embedded MATLAB Function1 ==
  data: u input double; y output double; T input double; f input double
function y = fcn(u,T,f)
% This block supports an embeddable subset of the MATLAB language.
% See the help menu for details. 

persistent a
persistent b
persistent y_km1
persistent u_km1
if isempty(a)
    %tf = [T*omega/(2+T*omega) T*omega/(2+T*omega)],[1 (T*omega-2)/(T*omega+2)]
    %tf = [a a],[1 -b]
    omega = 2*pi*f;
    a=T*omega/(2+T*omega);
    b=-(T*omega-2)/(T*omega+2);
    y_km1=u;
    u_km1=u;
end

y = a*(u+u_km1)+b*y_km1;
y_km1=y;
u_km1=u;

== matlab function Control Surface Input/myMux Fun5 ==
  data: u1 input double; y output double; u2 input double; u3 input double; u4 input double; u5 input double
function y = myMux(u1, u2, u3, u4, u5)
% This block supports an embeddable subset of the MATLAB language.
% See the help menu for details. 

y = [u1(1); u2(1); u3(1); u4(1); u5(1)];

== matlab function Sensor Data/Sensor Suite/If no HIL then Read all the Sensors/myMux Fun4 ==
  data: u1 input double; y output double; u2 input double; u3 input double; u4 input double; u5 input double; u6 input double; u7 input double; u8 input double; u9 input double; u10 input double; u11 input double; u12 input double; u13 input double
function y = sensMux(u1, u2,u3,u4,u5,u6,u7,u8, u9, u10, u11, u12, u13)
% This block supports an embeddable subset of the MATLAB language.
% See the help menu for details. 

y = [u1(1); u2(1); u3(1); u4(1); u5(1); u6(1); u7(1); u8(1); u9(1); u10(1); u11(1); u12(1); u13(1)];

== matlab function Sensor Data/Sensor Suite/If no HIL then Read all the Sensors/myMux Fun ==
  data: u1 input double; y output double; u2 input double; u3 input double; u4 input double
function y = myMux(u1, u2, u3, u4)
% This block supports an embeddable subset of the MATLAB language.
% See the help menu for details. 

y = [u1(1); u2(1); u3(1); u4(1)];

== matlab function Read Barometer BMP180/Baro Altimeter/Enables/Disables the Computation of initial Baro Bias ==
  data: tOut output double
function tOut = getTIni

persistent aveCount;
persistent tIni;

if isempty(aveCount)
    aveCount =1;
    tIni = 1;
end;

if aveCount < 2500
    aveCount = aveCount + 1;
end

if aveCount == 2500
    tIni =0;
    aveCount = aveCount + 1;
end

tOut = tIni;

%if aveCount > 500
%    tIni = 0;
%end

% if isempty(aveCount)
%     aveCount =1;
%     initBias = [0.0 0.0 0.0]';
% end;
%     
% if (aveCount<10)
%     initBias = initBias+ Raw;
%     bias = initBias/aveCount;
%     aveCount = aveCount +1;
% end;
% 
% if (aveCount == 10)
%     initBias = initBias/(aveCount-1);
%     aveCount = 100;
% end;
% 
% if (aveCount == 100)
%     bias = initBias;
% end;

== matlab function Sensor Data/Sensor Suite/ADIS16405 Signal Cond /3D Tustin Lowpass, Auto Initial Condition2/Embedded MATLAB Function2 ==
  data: u input double; y output double; T input double; f input double
function y = fcn(u,T,f)
% This block supports an embeddable subset of the MATLAB language.
% See the help menu for details. 

persistent a
persistent b
persistent y_km1
persistent u_km1
if isempty(a)
    %tf = [T*omega/(2+T*omega) T*omega/(2+T*omega)],[1 (T*omega-2)/(T*omega+2)]
    %tf = [a a],[1 -b]
    omega = 2*pi*f;
    a=T*omega/(2+T*omega);
    b=-(T*omega-2)/(T*omega+2);
    y_km1=u;
    u_km1=u;
end

y = a*(u+u_km1)+b*y_km1;
y_km1=y;
u_km1=u;

== matlab function Sensor Data/Sensor Suite/ADIS16405 Signal Cond /3D Tustin Lowpass, Auto Initial Condition2/myMux Fun ==
  data: u1 input double; y output double; u2 input double; u3 input double
function y = myMux3(u1, u2, u3)
% This block supports an embeddable subset of the MATLAB language.
% See the help menu for details. 

y = [u1(1); u2(1); u3(1)];

== matlab function Sensor Data/Sensor Suite/If no HIL then Read all the Sensors/Embedded MATLAB Function ==
  data: u input double; y output double
function y = averageADC(u)
% This block supports an embeddable subset of the MATLAB language.
% See the help menu for details. 

y = (u(1)+ u(2) + u(3) + u(4) + u(5))*0.20;

== matlab function Sensor Data/Sensor Suite/If no HIL then Read all the Sensors/Embedded MATLAB Function1 ==
  data: u input double; y output double
function y = averageADC(u)
% This block supports an embeddable subset of the MATLAB language.
% See the help menu for details. 

y = (u(1)+ u(2) + u(3) + u(4) + u(5))*0.20;

== matlab function Sensor Data/Sensor Suite/If no HIL then Read all the Sensors/Embedded MATLAB Function2 ==
  data: u input double; y output double
function y = averageADC(u)
% This block supports an embeddable subset of the MATLAB language.
% See the help menu for details. 

y = (u(1)+ u(2) + u(3) + u(4) + u(5))*0.20;

== matlab function Sensor Data/Sensor Suite/If no HIL then Read all the Sensors/Embedded MATLAB Function3 ==
  data: u input double; y output double
function y = averageADC(u)
% This block supports an embeddable subset of the MATLAB language.
% See the help menu for details. 

y = (u(1)+ u(2) + u(3) + u(4) + u(5))*0.20;

== matlab function Sensor Data/Sensor Suite/myMux Fun1 ==
  data: u1 input double; y output double; u2 input double; u3 input double; u4 input double
function y = myMux31(u1, u2, u3, u4)
% This block supports an embeddable subset of the MATLAB language.
% See the help menu for details. 

y = [u1(1); u2(1); u3(1); u4(1)];

== matlab function Sensor Data/Sensor Suite/ADIS16405 Signal Cond /3D Tustin Lowpass, Auto Initial Condition/Embedded MATLAB Function ==
  data: u input double; y output double; T input double; f input double
function y = fcn(u,T,f)
% This block supports an embeddable subset of the MATLAB language.
% See the help menu for details. 

persistent a
persistent b
persistent y_km1
persistent u_km1
if isempty(a)
    %tf = [T*omega/(2+T*omega) T*omega/(2+T*omega)],[1 (T*omega-2)/(T*omega+2)]
    %tf = [a a],[1 -b]
    omega = 2*pi*f;
    a=T*omega/(2+T*omega);
    b=-(T*omega-2)/(T*omega+2);
    y_km1=u;
    u_km1=u;
end

y = a*(u+u_km1)+b*y_km1;
y_km1=y;
u_km1=u;

== matlab function Sensor Data/Sensor Suite/ADIS16405 Signal Cond /3D Tustin Lowpass, Auto Initial Condition/Embedded MATLAB Function1 ==
  data: u input double; y output double; T input double; f input double
function y = fcn(u,T,f)
% This block supports an embeddable subset of the MATLAB language.
% See the help menu for details. 

persistent a
persistent b
persistent y_km1
persistent u_km1
if isempty(a)
    %tf = [T*omega/(2+T*omega) T*omega/(2+T*omega)],[1 (T*omega-2)/(T*omega+2)]
    %tf = [a a],[1 -b]
    omega = 2*pi*f;
    a=T*omega/(2+T*omega);
    b=-(T*omega-2)/(T*omega+2);
    y_km1=u;
    u_km1=u;
end

y = a*(u+u_km1)+b*y_km1;
y_km1=y;
u_km1=u;

== matlab function Sensor Data/Sensor Suite/ADIS16405 Signal Cond /3D Tustin Lowpass, Auto Initial Condition/Embedded MATLAB Function2 ==
  data: u input double; y output double; T input double; f input double
function y = fcn(u,T,f)
% This block supports an embeddable subset of the MATLAB language.
% See the help menu for details. 

persistent a
persistent b
persistent y_km1
persistent u_km1
if isempty(a)
    %tf = [T*omega/(2+T*omega) T*omega/(2+T*omega)],[1 (T*omega-2)/(T*omega+2)]
    %tf = [a a],[1 -b]
    omega = 2*pi*f;
    a=T*omega/(2+T*omega);
    b=-(T*omega-2)/(T*omega+2);
    y_km1=u;
    u_km1=u;
end

y = a*(u+u_km1)+b*y_km1;
y_km1=y;
u_km1=u;

== matlab function Sensor Data/Sensor Suite/ADIS16405 Signal Cond /3D Tustin Lowpass, Auto Initial Condition/myMux Fun ==
  data: u1 input double; y output double; u2 input double; u3 input double
function y = myMux3(u1, u2, u3)
% This block supports an embeddable subset of the MATLAB language.
% See the help menu for details. 

y = [u1(1); u2(1); u3(1)];

== matlab function Sensor Data/Sensor Suite/ADIS16405 Signal Cond /3D Tustin Lowpass, Auto Initial Condition1/Embedded MATLAB Function ==
  data: u input double; y output double; T input double; f input double
function y = fcn(u,T,f)
% This block supports an embeddable subset of the MATLAB language.
% See the help menu for details. 

persistent a
persistent b
persistent y_km1
persistent u_km1
if isempty(a)
    %tf = [T*omega/(2+T*omega) T*omega/(2+T*omega)],[1 (T*omega-2)/(T*omega+2)]
    %tf = [a a],[1 -b]
    omega = 2*pi*f;
    a=T*omega/(2+T*omega);
    b=-(T*omega-2)/(T*omega+2);
    y_km1=u;
    u_km1=u;
end

y = a*(u+u_km1)+b*y_km1;
y_km1=y;
u_km1=u;

== matlab function Sensor Data/Sensor Suite/ADIS16405 Signal Cond /3D Tustin Lowpass, Auto Initial Condition1/Embedded MATLAB Function1 ==
  data: u input double; y output double; T input double; f input double
function y = fcn(u,T,f)
% This block supports an embeddable subset of the MATLAB language.
% See the help menu for details. 

persistent a
persistent b
persistent y_km1
persistent u_km1
if isempty(a)
    %tf = [T*omega/(2+T*omega) T*omega/(2+T*omega)],[1 (T*omega-2)/(T*omega+2)]
    %tf = [a a],[1 -b]
    omega = 2*pi*f;
    a=T*omega/(2+T*omega);
    b=-(T*omega-2)/(T*omega+2);
    y_km1=u;
    u_km1=u;
end

y = a*(u+u_km1)+b*y_km1;
y_km1=y;
u_km1=u;

== matlab function Sensor Data/Sensor Suite/ADIS16405 Signal Cond /3D Tustin Lowpass, Auto Initial Condition1/Embedded MATLAB Function2 ==
  data: u input double; y output double; T input double; f input double
function y = fcn(u,T,f)
% This block supports an embeddable subset of the MATLAB language.
% See the help menu for details. 

persistent a
persistent b
persistent y_km1
persistent u_km1
if isempty(a)
    %tf = [T*omega/(2+T*omega) T*omega/(2+T*omega)],[1 (T*omega-2)/(T*omega+2)]
    %tf = [a a],[1 -b]
    omega = 2*pi*f;
    a=T*omega/(2+T*omega);
    b=-(T*omega-2)/(T*omega+2);
    y_km1=u;
    u_km1=u;
end

y = a*(u+u_km1)+b*y_km1;
y_km1=y;
u_km1=u;

== matlab function Sensor Data/Sensor Suite/ADIS16405 Signal Cond /3D Tustin Lowpass, Auto Initial Condition1/myMux Fun ==
  data: u1 input double; y output double; u2 input double; u3 input double
function y = myMux3(u1, u2, u3)
% This block supports an embeddable subset of the MATLAB language.
% See the help menu for details. 

y = [u1(1); u2(1); u3(1)];

== matlab function Sensor Data/Sensor Suite/Low Pass Filtering,Temperature Compensation and Calibration/Baro Altimeter/Enables/Disables the Computation of initial Baro Bias ==
  data: tOut output double
function tOut = getTIni

persistent aveCount;
persistent tIni;

if isempty(aveCount)
    aveCount =1;
    tIni = 1;
end;

if aveCount < 2500
    aveCount = aveCount + 1;
end

if aveCount == 2500
    tIni =0;
    aveCount = aveCount + 1;
end

tOut = tIni;

%if aveCount > 500
%    tIni = 0;
%end

% if isempty(aveCount)
%     aveCount =1;
%     initBias = [0.0 0.0 0.0]';
% end;
%     
% if (aveCount<10)
%     initBias = initBias+ Raw;
%     bias = initBias/aveCount;
%     aveCount = aveCount +1;
% end;
% 
% if (aveCount == 10)
%     initBias = initBias/(aveCount-1);
%     aveCount = 100;
% end;
% 
% if (aveCount == 100)
%     bias = initBias;
% end;

== matlab function Sensor Data/Sensor Suite/Low Pass Filtering,Temperature Compensation and Calibration/Tustin Lowpass, Auto Initial Condition1/Embedded MATLAB Function ==
  data: u input double; y output double; T input double; f input double
function y = fcn(u,T,f)
% This block supports an embeddable subset of the MATLAB language.
% See the help menu for details. 

persistent a
persistent b
persistent y_km1
persistent u_km1
if isempty(a)
    %tf = [T*omega/(2+T*omega) T*omega/(2+T*omega)],[1 (T*omega-2)/(T*omega+2)]
    %tf = [a a],[1 -b]
    omega = 2*pi*f;
    a=T*omega/(2+T*omega);
    b=-(T*omega-2)/(T*omega+2);
    y_km1=u;
    u_km1=u;
end

y = a*(u+u_km1)+b*y_km1;
y_km1=y;
u_km1=u;
